simulink model "trigo_test_tmp"  (Simulink 8.3)
settings: Solver=FixedStepDiscrete  StartTime=0.0  StopTime=10000.0  RelTol=1e-3
settings Model: Creator=scaife  LastModifiedBy=bourbouh  CovSFcnEnable=on  ExtModeAutoUpdateStatusClock=off
settings DataIOCC: SignalLoggingName=sigsOut
settings DebuggingCC: SaveWithParameterizedLinksMsg=none  SignalResolutionControl=TryResolveAllWithWarning  SolverPrmCheckMsg=none  MultiTaskDSMMsg=warning  MultiTaskCondExecSysMsg=none  FrameProcessingCompatibilityMsg=error  StateNameClashWarn=none  StrictBusMsg=None
settings HardwareCC: TargetUnknown=on
settings SFSimCC: SimParseCustomCode=off

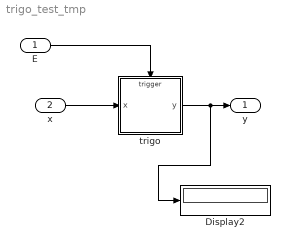
== system trigo_test_tmp ==
  E : Inport
  x : Inport  Port=2
  Display2 : Display
  trigo : Stateflow chart  TreatAsAtomicUnit=on
      settings: PermitHierarchicalResolution=ParametersOnly
  y : Outport
  wires:
  E/1 -> trigo/Trigger
  trigo/1(y) -> y/1, Display2/1
  x/1 -> trigo/1(x)

== stateflow chart trigo ==
  state A/
    en:y = cos(x);
  state B/
    en:y = sin(x);
  state C/
    en:y = tan(x);
  (default) -> A
  A -> B : E
  C -> A : E
  B -> C : E
  data: x input double; y output double
  events: E input RISING_EDGE_EVENT
